simulink model "RC_ckt"  (R2020b)
settings: Solver=VariableStepAuto  StartTime=0.0  StopTime=10  RelTol=1e-3
model workspace (MAT data in the model file):
  initial_values = 5
undefined symbols (not defined in the file): C, R
settings Model: Creator=shubham sharma  LastModifiedBy=shubham sharma

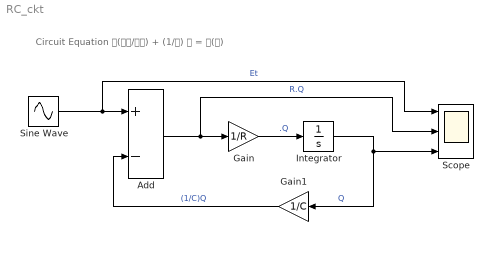
== system RC_ckt ==
  note: Circuit Equation
      | 𝑅(𝑑𝑄/𝑑𝑡) + (1/𝐶) 𝑄 = 𝐸(𝑡)
  Add : Sum  Inputs=+-
  Gain : Gain  Gain=1/R
  Gain1 : Gain  Gain=1/C
  Integrator : Integrator
  Scope : Scope  NumInputPorts=3
  Sine Wave : Sin  SampleTime=0
  wires:
  Sine Wave/1 -> Add/1, Scope/1  "Et"
  Add/1 -> Scope/2, Gain/1  "R.Q"
  Gain/1 -> Integrator/1  ".Q"
  Integrator/1 -> Scope/3, Gain1/1  "Q"
  Gain1/1 -> Add/2  "(1/C)Q"
